simulink model "AE3"  (R2015a)
settings: Solver=FixedStepDiscrete  SolverMode=SingleTasking  StartTime=0.0  StopTime=20  RelTol=1e-3
model workspace (MAT data in the model file):
  fa = 8000
  fsine = 1000
  spf = 1
libraries: dsparch4 x2, dspsrcs4 x2
settings Model: DataTypeOverride=Off  Creator=aluno  LastModifiedBy=aluno
settings DataIOCC: SaveOutput=off  SaveTime=off
settings OptimizationCC: BlockReduction=off  ConditionallyExecuteInputs=off  InlineParams=on
settings DebuggingCC: AlgebraicLoopMsg=error  SingleTaskRateTransMsg=error  StrictBusMsg=ErrorOnBusTreatedAsVector
settings HardwareCC: ProdHWDeviceType=ASIC/FPGA->ASIC/FPGA  ProdEqTarget=off

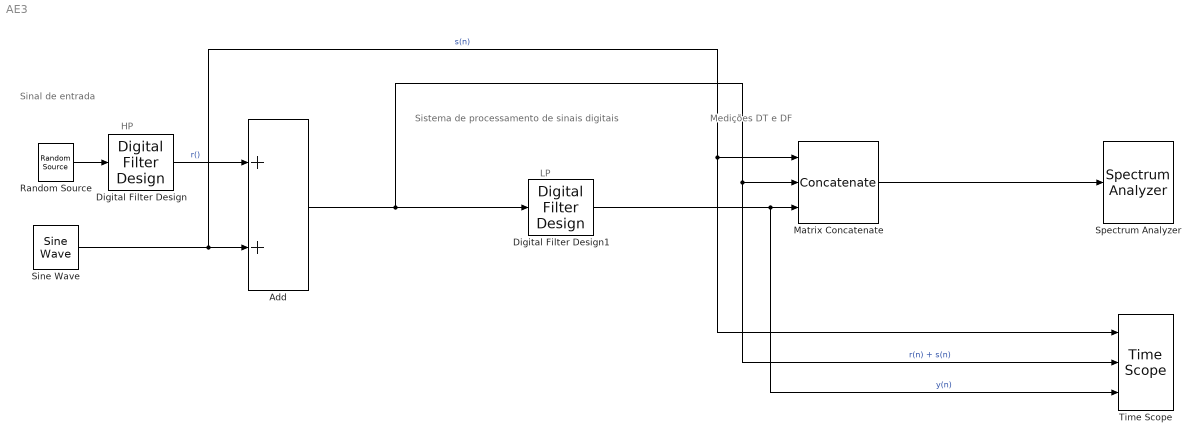
== system AE3 ==
  note: Medições DT e DF
  note: Sistema de processamento de sinais digitais
  note: Sinal de entrada
  note: LP
  note: HP
  Add : Sum
  Digital Filter Design : dsparch4/Digital Filter Design  mwdsp_browser_bugfix_var=off
  Digital Filter Design1 : dsparch4/Digital Filter Design  mwdsp_browser_bugfix_var=off
  Matrix Concatenate : Concatenate  NumInputs=3  Mode=Multidimensional array  ConcatenateDimension=2
  Random Source : dspsrcs4/Random Source  SrcType=Uniform  NormMethod=Ziggurat  CltLength=12  MinVal=0  MaxVal=5  MeanVal=0  VarVal=1  RepMode=Not repeatable  rawSeed=1  IsInherit=off  SampMode=Discrete  SampTime=1/fa  SampFrame=spf  DataType=Double  OutComplex=Real
  Sine Wave : dspsrcs4/Sine Wave  Amplitude=1  Frequency=fsine  Phase=0  SampleMode=Discrete  OutComplex=Real  CompMethod=Trigonometric fcn  TableSize=Memory  SampleTime=1/fa  SamplesPerFrame=spf  ResetState=Restart at time zero  dataType=double  wordLen=16  udDataType=sfix(16)  fracBitsMode=Best precision  numFracBits=15  OutDataTypeStr=double  LastOutDataTypeStr=double
  Spectrum Analyzer : SpectrumAnalyzer
  Time Scope : TimeScope  DefaultConfigurationName=spbscopes.TimeScopeBlockCfg  NumInputPorts=3
  wires:
  Random Source/1 -> Digital Filter Design/1
  Digital Filter Design/1 -> Add/1  "r()"
  Sine Wave/1 -> Time Scope/1, Matrix Concatenate/1, Add/2  "s(n)"
  Add/1 -> Digital Filter Design1/1, Time Scope/2, Matrix Concatenate/2  "r(n) + s(n)"
  Matrix Concatenate/1 -> Spectrum Analyzer/1
  Digital Filter Design1/1 -> Matrix Concatenate/3, Time Scope/3  "y(n)"
